simulink model "NL_Simulation"  (R2018b)
settings: Solver=VariableStepAuto  StartTime=0.0  StopTime=12.4  FixedStep=0.01
model workspace: external: MAT-File /home/abhineet/Research/Nonlinear_Model/Simulation_6dof/NL_Sim/setup_NL.mat (data not in the file)
values from neighbouring files (symbols this model uses):
  StateVals = SetInitial(Vinf,AeroType)    [setup_NL.m]
undefined symbols (not defined in the file or in its folder): AC, Mass
libraries: Tools_6dofSimulation x24, aerolibasang x3, dspmathops x3, shared6dofsys x2, shared6dof x2, aerolibatmos2 x1, sharedtransform x1, sharedutil x1
(part 1 of 2)
settings Model: SimulationMode=rapid-accelerator  Creator=abhineet  LastModifiedBy=abhineet
settings DataIOCC: ExternalInput=untitled.getElement('Throttle'),[]  InitialState=getstatestruct(Op_Pur)  SaveOutput=off  SignalLogging=off  DSMLogging=off  SaveTime=off
settings DebuggingCC: ReadBeforeWriteMsg=DisableAll  WriteAfterWriteMsg=DisableAll  WriteAfterReadMsg=DisableAll  MultiTaskDSMMsg=none  SignalLabelMismatchMsg=warning  LibraryContextMissingDiagnostic=none  StrictBusMsg=ErrorOnBusTreatedAsVector  NonBusSignalsTreatedAsBus=warning
settings ModelReferenceCC: UpdateModelReferenceTargets=IfOutOfDate
settings SFSimCC: SFSimEcho=off  SimUseLocalCustomCode=off
settings RTWCC: RTWUseLocalCustomCode=off

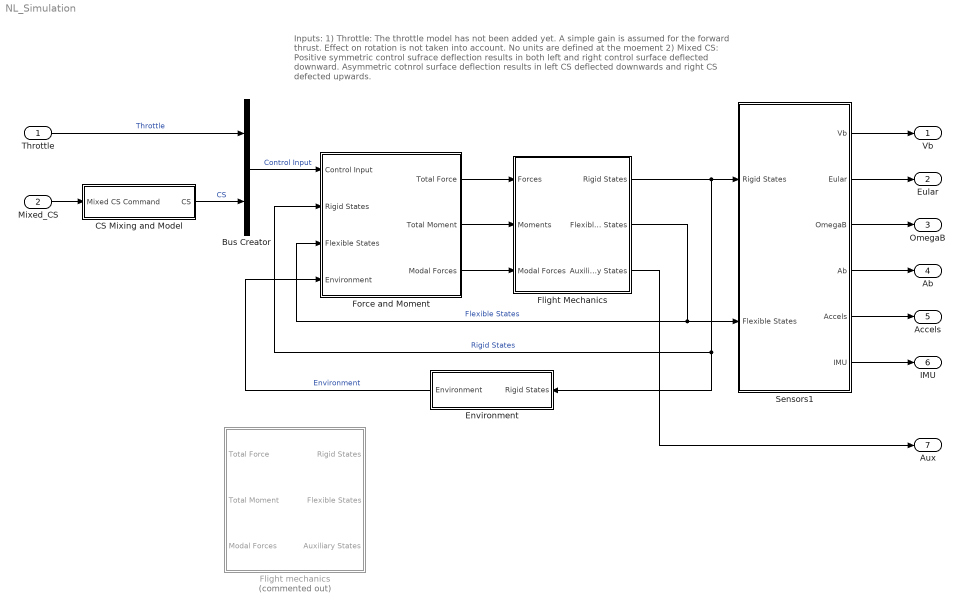
== system NL_Simulation ==
  note: Inputs:
      | 1) Throttle: The throttle model has not been added yet. A simple gain is assumed for the forward thrust.
      | 	Effect on rotation is not taken into account. No units are defined at the moement
      | 2) Mixed CS: Positive symmetric control sufrace deflection results in both left and right control surface
      | 	deflected downward. Asymmetric cotnrol surface deflection results in left CS deflected downwards
      | 	and right CS defected upwards.
  Throttle : Inport
  Mixed_CS : Inport  Port=2
  Bus Creator : BusCreator  Inputs=2
  CS Mixing and Model : Subsystem
  Environment : Subsystem
  Flight Mechanics : Subsystem  mask{units=Metric (MKS), xme_0=StateVals.Xe, Vm_0=StateVals.Vb, eul_0=StateVals.Eular, pm_0=StateVals.AngRates, mass_0=AC.MassProp.mass, inertia=AC.MassProp.inertia, xme_statename='', Vm_statename='', eul_statename='', pm_statename=''}
      mask prompts: xme_0 "Initial position in inertial axes [Xe,Ye,Ze]:"; Vm_0 "Initial velocity in body axes [U,v,w]:"; eul_0 "Initial Euler orientation [roll, pitch, yaw]:"; pm_0 "Initial body rotation rates [p,q,r]:"; mass_0 "Mass:"; xme_statename "Position: e.g., {'Xe', 'Ye', 'Ze'}"; Vm_statename "Velocity: e.g., {'U', 'v', 'w'}"; eul_statename "Euler roration angles: e.g., {'phi', 'theta', 'psi'}"; pm_statename "Body roration rates: e.g., {'p', 'q', 'r'}"
      mask TypeOptions units: Metric (MKS)
      mask DialogControl Container3 Prompt: State Names
  Flight mechanics : Subsystem  Commented=on
  "Force and Moment " : Subsystem
  Sensors1 : Subsystem
  Vb : Outport
  Eular : Outport  Port=2
  OmegaB : Outport  Port=3
  Ab : Outport  Port=4
  Accels : Outport  Port=5
  IMU : Outport  Port=6
  Aux : Outport  Port=7
  wires:
  "Force and Moment "/1(Total Force) -> Flight Mechanics/1(Forces)
  "Force and Moment "/2(Total Moment) -> Flight Mechanics/2(Moments)
  Bus Creator/1 -> "Force and Moment "/1(Control Input)  "Control Input"
  Flight Mechanics/1(Rigid States) -> Sensors1/1(Rigid States), "Force and Moment "/2(Rigid States), Environment/1(Rigid States)  "Rigid States"
  "Force and Moment "/3(Modal Forces) -> Flight Mechanics/3(Modal Forces)
  Flight Mechanics/2(Flexible States) -> Sensors1/2(Flexible States), "Force and Moment "/3(Flexible States)  "Flexible States"
  Environment/1(Environment) -> "Force and Moment "/4(Environment)  "Environment"
  CS Mixing and Model/1(CS) -> Bus Creator/2  "CS"
  Throttle/1 -> Bus Creator/1  "Throttle"
  Sensors1/3(OmegaB) -> OmegaB/1
  Sensors1/2(Eular) -> Eular/1
  Sensors1/4(Ab) -> Ab/1
  Sensors1/1(Vb) -> Vb/1
  Flight Mechanics/3(Auxiliary States) -> Aux/1
  Sensors1/6(IMU) -> IMU/1
  Sensors1/5(Accels) -> Accels/1
  Mixed_CS/1 -> CS Mixing and Model/1(Mixed CS Command)

== system NL_Simulation/CS Mixing and Model ==
  Mixed CS Command : Inport
  CS Mixing : Subsystem
  CS Model : Subsystem
  CS Model_old : Subsystem  Commented=on
  CS : Outport
  wires:
  CS Mixing/1(CS Command) -> CS Model/1(CS Command)
  CS Model/1(CS) -> CS/1
  Mixed CS Command/1 -> CS Mixing/1(Mixed CS Command)

== system NL_Simulation/Environment ==
  Rigid States : Inport
  Bus Creator : BusCreator  Inputs=1
  Bus Selector : BusSelector  OutputSignals=Xe
  COESA Atmosphere Model : aerolibatmos2/COESA Atmosphere Model  units=Metric (MKS)  spec=1976 COESA-extended U.S. Standard Atmosphere  model=Profile  profile_var=High temperature  profile_percent=1%  profile_alt=5 km (16404 ft)  envelope_var=High temperature  envelope_percent=1%  action=Warning
  Demux : Demux  Outputs=3
  Gain : Gain  Gain=-1
  Terminator{,1..4} (5 alike) : Terminator
  Environment : Outport
  wires:
  Rigid States/1 -> Bus Selector/1
  COESA Atmosphere Model/1 -> Terminator2/1
  COESA Atmosphere Model/2 -> Terminator1/1
  COESA Atmosphere Model/3 -> Terminator/1
  COESA Atmosphere Model/4 -> Bus Creator/1  "Rho"
  Bus Creator/1 -> Environment/1  "Environment"
  Bus Selector/1 -> Demux/1  "<Xe>"
  Demux/2 -> Terminator3/1
  Demux/1 -> Terminator4/1
  Demux/3 -> Gain/1  "Ze"
  Gain/1 -> COESA Atmosphere Model/1

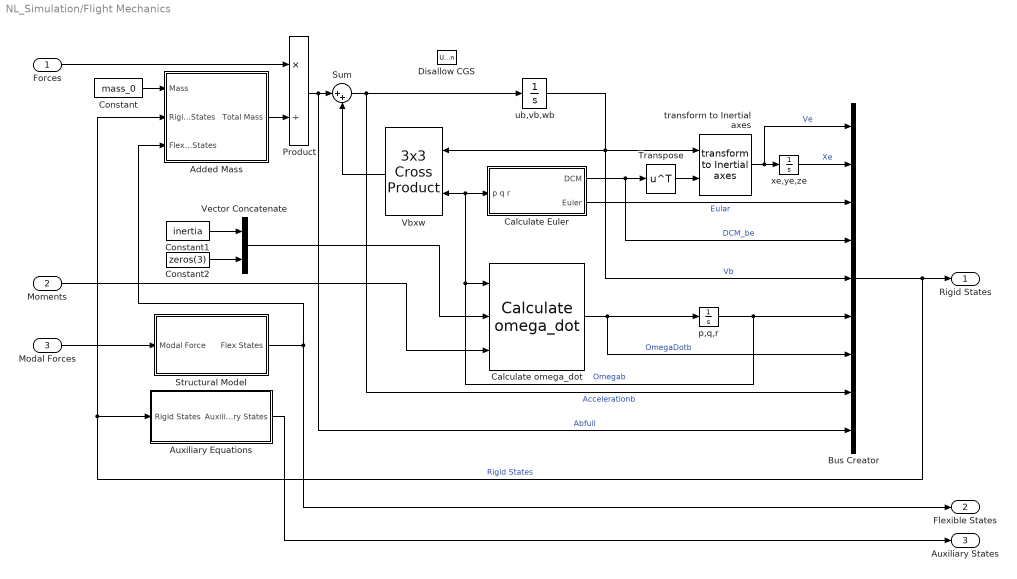
== system NL_Simulation/Flight Mechanics ==
  Forces : Inport  Unit=N  PortDimensions=3
  Moments : Inport  Port=2  Unit=N*m  PortDimensions=3
  Modal Forces : Inport  Port=3  Unit=N*m
  Added Mass : Subsystem
  "Auxiliary Equations " : Subsystem
  Bus Creator : BusCreator  Inputs=9
  Calculate Euler : Subsystem
  Calculate omega_dot : shared6dofsys/Calculate omega_dot  aMode=aMode
      settings: SourceProductName=Aerospace Blockset  SourceProductBaseCode=AE
  Constant : Constant  Value=mass_0  OutDataTypeStr=Inherit: Inherit via back propagation
  Constant1 : Constant  Value=inertia  OutDataTypeStr=Inherit: Inherit via back propagation
  Constant2 : Constant  Value=zeros(3)
  Disallow CGS : UnitConfiguration  UnitSystemsStr=English,SI,SI (extended)  AllowAllUnitSystems=off
  Product : Product  Inputs=*/  SaturateOnIntegerOverflow=on  OutDataTypeStr=Inherit: Same as first input
  Structural Model : Subsystem
  Sum : Sum  Inputs=|++  SaturateOnIntegerOverflow=on
  Transpose : Math  Operator=transpose  SaturateOnIntegerOverflow=on
  Vbxw : sharedutil/3x3 Cross Product  aMode=aMode
      settings: SourceProductBaseCode=AE
  Vector Concatenate : Concatenate  Mode=Multidimensional array
  "p,q,r " : Integrator  InitialCondition=pm_0  ContinuousStateAttributes=pm_statename
  "transform to Inertial axes " : shared6dof/6DOF (Euler Angles)/transform to Inertial axes   SystemSampleTime=-1
      settings: SourceProductName=Aerospace Blockset  SourceProductBaseCode=AE
  ub,vb,wb : Integrator  InitialCondition=Vm_0  ContinuousStateAttributes=Vm_statename
  xe,ye,ze : Integrator  InitialCondition=xme_0  ContinuousStateAttributes=xme_statename
  Rigid States : Outport
  Flexible States : Outport  Port=2
  Auxiliary States : Outport  Port=3
  wires:
  Constant/1 -> Added Mass/1(Mass)
  Vbxw/1 -> Sum/2
  Vector Concatenate/1 -> Calculate omega_dot/2
  Forces/1 -> Product/1
  Product/1 -> Bus Creator/9, Sum/1  "Abfull"
  Transpose/1 -> "transform to Inertial axes "/2
  Moments/1 -> Calculate omega_dot/3
  Added Mass/1(Total Mass) -> Product/2
  "transform to Inertial axes "/1 -> Bus Creator/1, xe,ye,ze/1  "Ve"
  xe,ye,ze/1 -> Bus Creator/2  "Xe"
  "p,q,r "/1 -> Calculate Euler/1("p q r "), Vbxw/2, Calculate omega_dot/1, Bus Creator/6  "Omegab"
  Calculate Euler/2(Euler) -> Bus Creator/3  "Eular"
  ub,vb,wb/1 -> Bus Creator/5, Vbxw/1, "transform to Inertial axes "/1  "Vb"
  Calculate Euler/1(DCM) -> Bus Creator/4, Transpose/1  "DCM_be"
  Calculate omega_dot/1 -> "p,q,r "/1, Bus Creator/7  "OmegaDotb"
  Sum/1 -> ub,vb,wb/1, Bus Creator/8  "Accelerationb"
  Bus Creator/1 -> Rigid States/1, "Auxiliary Equations "/1(Rigid States), Added Mass/2(Rigid States)  "Rigid States"
  Modal Forces/1 -> Structural Model/1(Modal Force)
  Structural Model/1(Flex States) -> Flexible States/1, Added Mass/3(Flexible States)
  Constant2/1 -> Vector Concatenate/2
  Constant1/1 -> Vector Concatenate/1
  "Auxiliary Equations "/1(Auxiliary States) -> Auxiliary States/1

== system NL_Simulation/Flight mechanics ==
  Total Force : Inport
  Total Moment : Inport  Port=2
  Modal Forces : Inport  Port=3
  "Auxiliary Equations " : Subsystem
  Subsystem1 : Subsystem  Commented=on
  Subsystem2 : Subsystem  Commented=on
  Rigid States : Outport
  Flexible States : Outport  Port=2
  Auxiliary States : Outport  Port=3
  wires:
  Total Moment/1 -> ?
  Total Force/1 -> ?
  ? -> "Auxiliary Equations "/1(Rigid States), Rigid States/1
  "Auxiliary Equations "/1(Auxiliary States) -> Auxiliary States/1
  Modal Forces/1 -> ?
  ? -> Flexible States/1

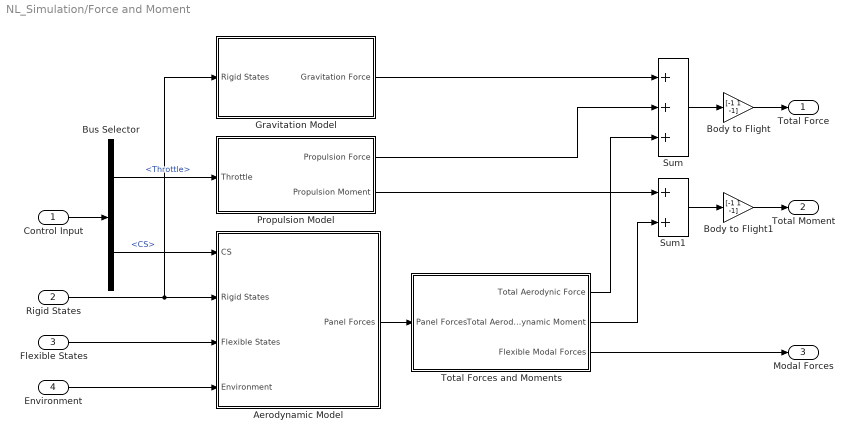
== system NL_Simulation/Force and Moment  ==
  Control Input : Inport
  Rigid States : Inport  Port=2
  Flexible States : Inport  Port=3
  Environment : Inport  Port=4
  Aerodynamic Model : Subsystem
  Body to Flight : Gain  Gain=[-1 1 -1]
  Body to Flight1 : Gain  Gain=[-1 1 -1]
  Bus Selector : BusSelector  OutputSignals=Throttle,CS
  Gravitation Model : Subsystem
  Propulsion Model : Subsystem
  Sum : Sum  Inputs=+++
  Sum1 : Sum
  Total Forces and Moments : Subsystem
  Total Force : Outport
  Total Moment : Outport  Port=2
  Modal Forces : Outport  Port=3
  wires:
  Control Input/1 -> Bus Selector/1
  Bus Selector/1 -> Propulsion Model/1(Throttle)  "<Throttle>"
  Bus Selector/2 -> Aerodynamic Model/1(CS)  "<CS>"
  Rigid States/1 -> Aerodynamic Model/2(Rigid States), Gravitation Model/1(Rigid States)
  Flexible States/1 -> Aerodynamic Model/3(" Flexible States")
  Sum/1 -> Body to Flight/1
  Environment/1 -> Aerodynamic Model/4(Environment)
  Total Forces and Moments/1(Total Aerodynic Force) -> Sum/3
  Total Forces and Moments/2(Total Aerodynamic Moment) -> Sum1/2
  Aerodynamic Model/1(Panel Forces) -> Total Forces and Moments/1(Panel Forces)
  Propulsion Model/1(Propulsion Force) -> Sum/2
  Gravitation Model/1(Gravitation Force) -> Sum/1
  Propulsion Model/2(Propulsion Moment) -> Sum1/1
  Sum1/1 -> Body to Flight1/1
  Body to Flight/1 -> Total Force/1
  Body to Flight1/1 -> Total Moment/1
  Total Forces and Moments/3(Flexible Modal Forces) -> Modal Forces/1

== system NL_Simulation/Sensors1 ==
  Rigid States : Inport
  Flexible States : Inport  Port=2
  Accelerometer Rigid : Subsystem  Commented=on
  Accelerometers : Subsystem
  Bus Selector : BusSelector  OutputSignals=Vb,Eular,Omegab,Accelerationb
  IMUs : Subsystem
  Sensors : Subsystem  Commented=on
  Vb : Outport
  Eular : Outport  Port=2
  OmegaB : Outport  Port=3
  Ab : Outport  Port=4
  Accels : Outport  Port=5
  IMU : Outport  Port=6
  wires:
  Rigid States/1 -> IMUs/1(Rigid States), Accelerometers/1(Rigid States), Bus Selector/1
  Flexible States/1 -> IMUs/2(Flexible States), Accelerometers/2(Flexible States)
  Bus Selector/3 -> OmegaB/1  "<Omegab>"
  Bus Selector/2 -> Eular/1  "<Eular>"
  Bus Selector/4 -> Ab/1  "<Accelerationb>"
  Bus Selector/1 -> Vb/1  "<Vb>"
  Accelerometers/1(Accels) -> Accels/1
  IMUs/1(IMU) -> IMU/1

== system NL_Simulation/CS Mixing and Model/CS Mixing ==
  Mixed CS Command : Inport
  Demux : Demux  Outputs=8
  Mux : Mux  Inputs=8
  Sum{,1..3} (4 alike) : Sum  Inputs=|++
  Sum{4..7} (4 alike) : Sum  Inputs=+-|
  CS Command : Outport
  wires:
  Demux/7 -> Sum6/2, Sum2/2  "Asym 3"
  Sum/1 -> Mux/1  "L1"
  Sum4/1 -> Mux/5  "R1"
  Sum7/1 -> Mux/8  "R4"
  Demux/8 -> Sum7/2, Sum3/2  "Asym 4"
  Demux/2 -> Sum5/1, Sum1/1  "Sym 2"
  Demux/1 -> Sum4/1, Sum/1  "Sym 1"
  Demux/4 -> Sum7/1, Sum3/1  "Sym 4"
  Sum1/1 -> Mux/2  "L2"
  Demux/5 -> Sum4/2, Sum/2  "Asym 1"
  Sum2/1 -> Mux/3  "L3"
  Demux/3 -> Sum6/1, Sum2/1  "Sym 3"
  Sum5/1 -> Mux/6  "R2"
  Sum6/1 -> Mux/7  "R3"
  Demux/6 -> Sum5/2, Sum1/2  "Asym 2"
  Mixed CS Command/1 -> Demux/1
  Sum3/1 -> Mux/4  "L4"
  Mux/1 -> CS Command/1

== system NL_Simulation/CS Mixing and Model/CS Model ==
  note: A second order actuator model is used: b/(s^2 + as + b)
  CS Command : Inport
  Actuator_a : Gain  Gain=AC.Actuator.a
  Actuator_b : Gain  Gain=AC.Actuator.b
  Bus Creator : BusCreator  Inputs=2
  CS Pos : Integrator  InitialCondition=StateVals.CSPos
  CS Vel : Integrator  InitialCondition=StateVals.CSVel
  Scope : Scope
  Sum : Sum  Inputs=|+-
  Sum1 : Sum  Inputs=|+-
  CS : Outport
  wires:
  CS Pos/1 -> Sum/2, Bus Creator/1  "CS Pos"
  CS Vel/1 -> Scope/1, CS Pos/1, Actuator_a/1, Bus Creator/2  "CS Vel"
  Actuator_b/1 -> Sum1/1
  CS Command/1 -> Sum/1
  Sum/1 -> Actuator_b/1
  Actuator_a/1 -> Sum1/2
  Sum1/1 -> CS Vel/1
  Bus Creator/1 -> CS/1

== system NL_Simulation/CS Mixing and Model/CS Model_old ==
  CS Command : Inport
  Bus Creator : BusCreator  Inputs=2
  CS Pos : Integrator  InitialCondition=StateVals.CSPos
  Gain : Gain  Gain=AC.CS.CSTau
  Sum : Sum  Inputs=|+-
  CS : Outport
  wires:
  CS Command/1 -> Sum/1
  Sum/1 -> Gain/1
  Gain/1 -> Bus Creator/2, CS Pos/1  "CS Vel"
  CS Pos/1 -> Bus Creator/1, Sum/2  "CS Pos"
  Bus Creator/1 -> CS/1  "CS"

== system NL_Simulation/Flight Mechanics/Added Mass ==
  Mass : Inport
  Rigid States : Inport  Port=2
  Flexible States : Inport  Port=3
  Mux : Mux  Inputs=3
  Subsystem3 : Subsystem  Commented=on
  Sum1 : Sum
  Sum2 : Sum
  Sum3 : Sum
  Total Mass : Outport
  wires:
  Mass/1 -> Sum3/1, Sum2/1, Sum1/1
  Subsystem3/1(Mx) -> Sum1/2
  Subsystem3/2(My) -> Sum2/2
  Subsystem3/3(Mz) -> Sum3/2
  Sum1/1 -> Mux/1
  Sum2/1 -> Mux/2
  Sum3/1 -> Mux/3
  Mux/1 -> Total Mass/1
  Rigid States/1 -> Subsystem3/1(Rigid States)
  Flexible States/1 -> Subsystem3/2(Flexible States)

== system NL_Simulation/Flight Mechanics/Auxiliary Equations  ==
  Rigid States : Inport
  Bus Creator1 : BusCreator  Inputs=3
  Bus Selector : BusSelector  OutputSignals=Vb
  "Incidence, Sideslip, & Airspeed" : aerolibasang/Incidence, Sideslip, & Airspeed
      settings: SourceProductName=Aerospace Blockset
  Auxiliary States : Outport
  wires:
  Bus Creator1/1 -> Auxiliary States/1  "Wind Parameters"
  "Incidence, Sideslip, & Airspeed"/3 -> Bus Creator1/3  "vinf"
  "Incidence, Sideslip, & Airspeed"/2 -> Bus Creator1/2  "beta"
  "Incidence, Sideslip, & Airspeed"/1 -> Bus Creator1/1  "alpha"
  Rigid States/1 -> Bus Selector/1  "Rigid States"
  Bus Selector/1 -> "Incidence, Sideslip, & Airspeed"/1  "<Vb>"

== system NL_Simulation/Flight Mechanics/Calculate Euler ==
  "p q r " : Inport
  Rotation Angles to Direction Cosine Matrix : sharedtransform/Rotation Angles to Direction Cosine Matrix  rotationOrder=ZYX  aMode=aMode
      settings: SourceProductBaseCode=AE
  Selector : Selector  InputPortWidth=3  IndexOptions=Index vector (dialog)  Indices=[3 2 1]  OutputSizes=1
  phi theta psi : Integrator  InitialCondition=eul_0  WrapState=on  ContinuousStateAttributes=eul_statename
  phidot thetadot psidot : shared6dofsys/DCM & Euler Angles (Euler)/phidot thetadot psidot  SystemSampleTime=-1
      settings: SourceProductName=Aerospace Blockset  SourceProductBaseCode=AE
  DCM : Outport
  Euler : Outport  Port=2
  wires:
  phidot thetadot psidot/1 -> phi theta psi/1
  "p q r "/1 -> phidot thetadot psidot/1
  phi theta psi/1 -> Selector/1, phidot thetadot psidot/2, Euler/1
  Rotation Angles to Direction Cosine Matrix/1 -> DCM/1
  Selector/1 -> Rotation Angles to Direction Cosine Matrix/1

== system NL_Simulation/Flight Mechanics/Structural Model ==
  Modal Force : Inport
  Bus Creator : BusCreator  Inputs=3
  Damping : Gain  Gain=AC.ModalStruc.Damping
  Eta : Integrator  InitialCondition=StateVals.Eta
  Etadot : Integrator  InitialCondition=StateVals.EtaDot
  InverseMass : Gain  Gain=AC.ModalStruc.InvMass
  Stiffness : Gain  Gain=AC.ModalStruc.Stiffness
  Sum : Sum  Inputs=|+-
  Sum1 : Sum  Inputs=|+-
  Flex States : Outport
  wires:
  InverseMass/1 -> Bus Creator/3, Etadot/1  "EtaFlexdotdot"
  Etadot/1 -> Damping/1, Bus Creator/2, Eta/1  "EtaFlexdot"
  Damping/1 -> Sum/2
  Eta/1 -> Bus Creator/1, Stiffness/1  "EtaFlex"
  Sum/1 -> InverseMass/1
  Sum1/1 -> Sum/1
  Modal Force/1 -> Sum1/1
  Bus Creator/1 -> Flex States/1  "Flex States"
  Stiffness/1 -> Sum1/2

== system NL_Simulation/Flight mechanics/Auxiliary Equations  ==
  Rigid States : Inport
  Bus Creator1 : BusCreator  Inputs=3
  Bus Selector : BusSelector  OutputSignals=Vb
  "Incidence, Sideslip, & Airspeed" : aerolibasang/Incidence, Sideslip, & Airspeed
      settings: SourceProductName=Aerospace Blockset
  Auxiliary States : Outport
  wires:
  Bus Creator1/1 -> Auxiliary States/1  "Wind Parameters"
  "Incidence, Sideslip, & Airspeed"/3 -> Bus Creator1/3  "vinf"
  "Incidence, Sideslip, & Airspeed"/2 -> Bus Creator1/2  "beta"
  "Incidence, Sideslip, & Airspeed"/1 -> Bus Creator1/1  "alpha"
  Rigid States/1 -> Bus Selector/1  "Rigid States"
  Bus Selector/1 -> "Incidence, Sideslip, & Airspeed"/1  "<Vb>"

== system NL_Simulation/Flight mechanics/Subsystem1 ==
  In1 : Inport
  In2 : Inport  Port=2
  In3 : Inport  Port=3
  6DOF : shared6dof/6DOF (Euler Angles)  units=Metric (MKS)  mtype=Fixed  rep=Euler Angles  xme_0=StateVals.Xe  Vm_0=StateVals.Vb  eul_0=StateVals.Eular  pm_0=StateVals.AngRates  mass_0=AC.MassProp.mass  mass_e=0.5  mass_f=2.0  inertia=AC.MassProp.inertia  inertia_e=eye(3)  inertia_f=2*eye(3)  k_quat=1.0  vre_flag=on  abi_flag=off  aMode=0  xme_statename=''  Vm_statename=''  eul_statename=''  quat_statename=''  pm_statename=''  mass_statename=''
      settings: SourceProductBaseCode=AE
  "Auxiliary Equations " : Subsystem
  Bus Creator : BusCreator  Inputs=8
  Structural Model : Subsystem
  Rigid States : Outport
  Flexible States : Outport  Port=2
  Auxiliary States : Outport  Port=3
  wires:
  6DOF/3 -> Bus Creator/3  "Eular"
  "Auxiliary Equations "/1(Auxiliary States) -> Auxiliary States/1
  6DOF/4 -> Bus Creator/4  "DCM_be"
  6DOF/5 -> Bus Creator/5  "Vb"
  6DOF/6 -> Bus Creator/6  "Omegab"
  In1/1 -> 6DOF/1
  In2/1 -> 6DOF/2
  In3/1 -> Structural Model/1(Modal Force)
  Bus Creator/1 -> Rigid States/1, "Auxiliary Equations "/1(Rigid States)  "Rigid States"
  Structural Model/1(Flex States) -> Flexible States/1
  6DOF/2 -> Bus Creator/2  "Xe"
  6DOF/1 -> Bus Creator/1  "Ve"
  6DOF/7 -> Bus Creator/7  "OmegaDotb"
  6DOF/8 -> Bus Creator/8  "Accelerationb"

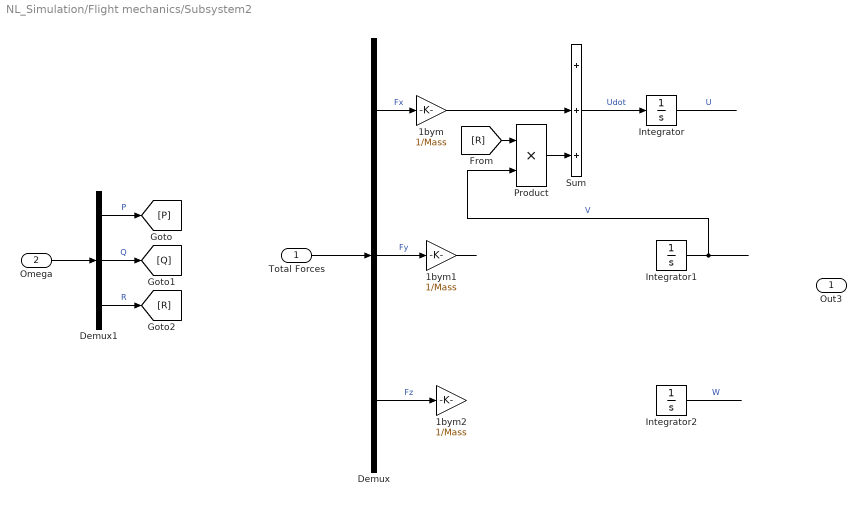
== system NL_Simulation/Flight mechanics/Subsystem2 ==
  Total Forces : Inport
  Omega : Inport  Port=2
  1bym : Gain  Gain=1/Mass
  1bym1 : Gain  Gain=1/Mass
  1bym2 : Gain  Gain=1/Mass
  Demux : Demux  Outputs=3
  Demux1 : Demux  Outputs=3
  Integrator : Integrator
  Integrator1 : Integrator
  Integrator2 : Integrator
  Product : Product
  Sum : Sum  Inputs=+++
  Out3 : Outport
  wires:
  Product/1 -> Sum/3
  1bym1/1 -> ?
  Demux/1 -> 1bym/1  "Fx"
  Demux1/3 -> [R]  "R"
  Omega/1 -> Demux1/1
  Demux/2 -> 1bym1/1  "Fy"
  Integrator/1 -> ?  "U"
  Demux1/2 -> [Q]  "Q"
  Total Forces/1 -> Demux/1
  1bym/1 -> Sum/2
  Demux1/1 -> [P]  "P"
  Sum/1 -> Integrator/1  "Udot"
  Demux/3 -> 1bym2/1  "Fz"
  Integrator1/1 -> Product/2  "V"
  ? -> Integrator1/1  "Vdot"
  ? -> Integrator2/1  "Wdot"
  Integrator2/1 -> ?  "W"
  [R] -> Product/1

== system NL_Simulation/Force and Moment /Aerodynamic Model ==
  CS : Inport
  Rigid States : Inport  Port=2
  " Flexible States" : Inport  Port=3
  Environment : Inport  Port=4
  Steady Aerodynamics : Subsystem
  Sum : Sum
  Unsteady Aerodynamics : Subsystem  Commented=on
  Panel Forces : Outport
  wires:
  CS/1 -> Steady Aerodynamics/1(CS)
  Rigid States/1 -> Unsteady Aerodynamics/1(Rigid States), Steady Aerodynamics/2(Rigid States)
  " Flexible States"/1 -> Unsteady Aerodynamics/2(Flexible States), Steady Aerodynamics/3(Flexible States)
  Environment/1 -> Steady Aerodynamics/4(Environment)
  Steady Aerodynamics/1(Total Steady Forces) -> Sum/1
  Sum/1 -> Panel Forces/1
  Unsteady Aerodynamics/1(Total Unsteady Forces) -> Sum/2

== system NL_Simulation/Force and Moment /Gravitation Model ==
  note: Gravitational force is first calculated in body fixed, flight dynamics axes and then converted to Aerodynamic Axes
  Rigid States : Inport
  Bus Selector : BusSelector  OutputSignals=DCM_be
  Constant : Constant  Value=0
  Flight Dynamics to Aero Axes : Gain  Gain=[-1 1 -1]
  Mass : Constant  Value=AC.MassProp.mass
  Mux : Mux  Inputs=3
  Product1 : Product
  Product2 : Product  Multiplication=Matrix(*)
  Reshape : Reshape  OutputDimensionality=Column vector (2-D)
  Reshape1 : Reshape
  g : Constant  Value=9.81
  Gravitation Force : Outport
  wires:
  Rigid States/1 -> Bus Selector/1
  Bus Selector/1 -> Product2/1  "<DCM_be>"
  Mass/1 -> Product1/2
  g/1 -> Product1/1
  Flight Dynamics to Aero Axes/1 -> Gravitation Force/1
  Product2/1 -> Reshape1/1
  Constant/1 -> Mux/2, Mux/1
  Product1/1 -> Mux/3  "mg"
  Mux/1 -> Reshape/1
  Reshape/1 -> Product2/2
  Reshape1/1 -> Flight Dynamics to Aero Axes/1

== system NL_Simulation/Force and Moment /Propulsion Model ==
  note: Propulsion forces and moments are calculated in Aerodynamic Axes directly
  Throttle : Inport
  Gain : Gain  Gain=[-100 0 0]
  Gain1 : Gain  Gain=[0 0 0]
  Propulsion Force : Outport
  Propulsion Moment : Outport  Port=2
  wires:
  Gain/1 -> Propulsion Force/1
  Throttle/1 -> Gain1/1, Gain/1
  Gain1/1 -> Propulsion Moment/1

== system NL_Simulation/Force and Moment /Total Forces and Moments ==
  Panel Forces : Inport
  Constant1 : Constant  Value=AC.Aero.VLMData.grid.r_cgvortex
  MATLAB Function : MATLAB Function  TreatAsAtomicUnit=on
  RB Mode Tranlation : Gain  Gain=AC.ModalStruc.Phif_aero_trans'  Multiplication=Matrix(K*u)
  Reshape : Reshape
  Reshape1 : Reshape
  Sum : Sum  Inputs=+  CollapseMode=Specified dimension  CollapseDim=2
  Total Aerodynic Force : Outport
  Total Aerodynamic Moment : Outport  Port=2
  Flexible Modal Forces : Outport  Port=3
  wires:
  MATLAB Function/1(SumRcrossF) -> Total Aerodynamic Moment/1
  RB Mode Tranlation/1 -> Flexible Modal Forces/1
  Reshape/1 -> RB Mode Tranlation/1
  Panel Forces/1 -> Reshape/1, MATLAB Function/2(F), Sum/1
  Constant1/1 -> MATLAB Function/1(R)
  Sum/1 -> Reshape1/1
  Reshape1/1 -> Total Aerodynic Force/1

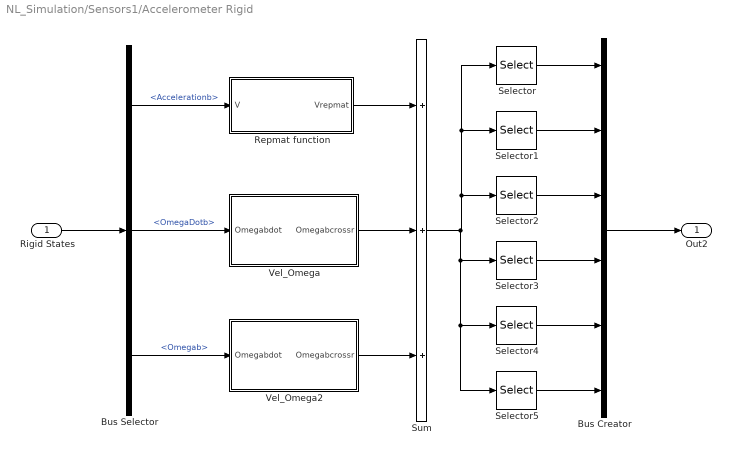
== system NL_Simulation/Sensors1/Accelerometer Rigid ==
  Rigid States : Inport
  Bus Creator : BusCreator  Inputs=6
  Bus Selector : BusSelector  OutputSignals=Accelerationb,OmegaDotb,Omegab
  Repmat function : MATLAB Function  TreatAsAtomicUnit=on  mask{NumSensors=AC.SensorData.NumSensors}
      mask prompts: NumSensors "Number of Sensors"
      mask init:
      | % NumPanels = 888;
  Selector : Selector  NumberOfDimensions=2  InputPortWidth=2  IndexOptions=Index vector (dialog),Index vector (dialog)  Indices=3,1  OutputSizes=1,1
  Selector1 : Selector  NumberOfDimensions=2  InputPortWidth=2  IndexOptions=Index vector (dialog),Index vector (dialog)  Indices=3,2  OutputSizes=1,1
  Selector2 : Selector  NumberOfDimensions=2  InputPortWidth=2  IndexOptions=Index vector (dialog),Index vector (dialog)  Indices=3,3  OutputSizes=1,1
  Selector3 : Selector  NumberOfDimensions=2  InputPortWidth=2  IndexOptions=Index vector (dialog),Index vector (dialog)  Indices=3,4  OutputSizes=1,1
  Selector4 : Selector  NumberOfDimensions=2  InputPortWidth=2  IndexOptions=Index vector (dialog),Index vector (dialog)  Indices=3,5  OutputSizes=1,1
  Selector5 : Selector  NumberOfDimensions=2  InputPortWidth=2  IndexOptions=Index vector (dialog),Index vector (dialog)  Indices=3,6  OutputSizes=1,1
  Sum : Sum  Inputs=+++
  Vel_Omega : Subsystem
  Vel_Omega2 : Subsystem
  Out2 : Outport
  wires:
  Rigid States/1 -> Bus Selector/1
  Bus Selector/1 -> Repmat function/1(V)  "<Accelerationb>"
  Bus Selector/2 -> Vel_Omega/1(Omegabdot)  "<OmegaDotb>"
  Vel_Omega/1(Omegabcrossr) -> Sum/2
  Repmat function/1(Vrepmat) -> Sum/1
  Bus Selector/3 -> Vel_Omega2/1(Omegabdot)  "<Omegab>"
  Vel_Omega2/1(Omegabcrossr) -> Sum/3
  Sum/1 -> Selector4/1, Selector5/1, Selector3/1, Selector/1, Selector1/1, Selector2/1
  Selector/1 -> Bus Creator/1
  Selector1/1 -> Bus Creator/2
  Selector2/1 -> Bus Creator/3
  Selector3/1 -> Bus Creator/4
  Selector5/1 -> Bus Creator/6
  Selector4/1 -> Bus Creator/5
  Bus Creator/1 -> Out2/1

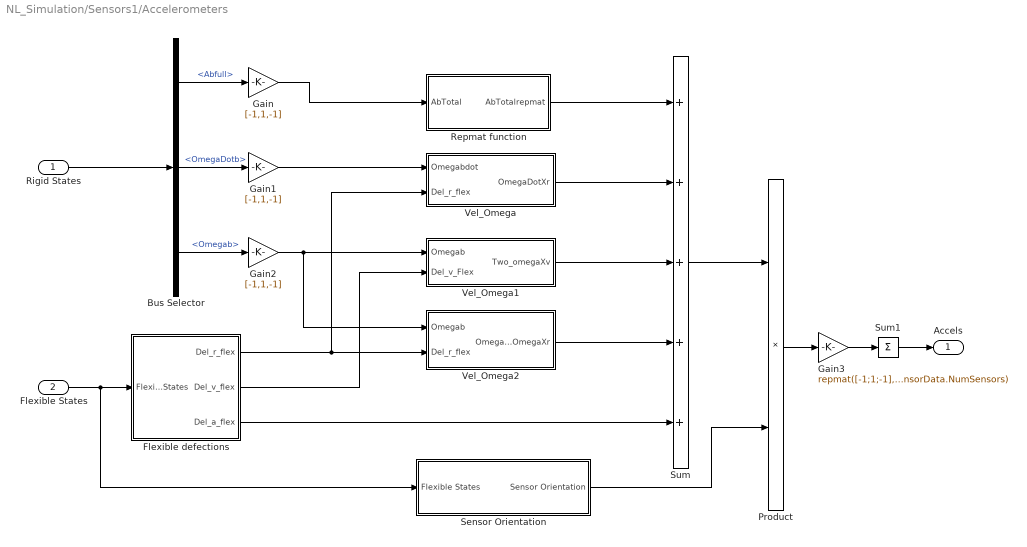
== system NL_Simulation/Sensors1/Accelerometers ==
  Rigid States : Inport
  Flexible States : Inport  Port=2
  Bus Selector : BusSelector  OutputSignals=Abfull,OmegaDotb,Omegab
  Flexible defections : Subsystem
  Gain : Gain  Gain=[-1,1,-1]
  Gain1 : Gain  Gain=[-1,1,-1]
  Gain2 : Gain  Gain=[-1,1,-1]
  Gain3 : Gain  Gain=repmat([-1;1;-1],1,AC.SensorData.NumSensors)
  Product : Product
  Repmat function : MATLAB Function  TreatAsAtomicUnit=on  mask{NumSensors=AC.SensorData.NumSensors}
      mask prompts: NumSensors "Number of Sensors"
      mask init:
      | % NumPanels = 888;
  Sensor Orientation : Subsystem
  Sum : Sum  Inputs=+++++
  Sum1 : Sum  Inputs=+  CollapseMode=Specified dimension
  Vel_Omega : Subsystem
  Vel_Omega1 : Subsystem
  Vel_Omega2 : Subsystem
  Accels : Outport
  wires:
  Rigid States/1 -> Bus Selector/1
  Bus Selector/1 -> Gain/1  "<Abfull>"
  Vel_Omega/1(OmegaDotXr) -> Sum/2
  Vel_Omega2/1(OmegaXOmegaXr) -> Sum/4
  Flexible States/1 -> Sensor Orientation/1(Flexible States), Flexible defections/1(Flexible States)
  Sensor Orientation/1(Sensor Orientation) -> Product/2
  Product/1 -> Gain3/1
  Sum/1 -> Product/1
  Sum1/1 -> Accels/1
  Bus Selector/2 -> Gain1/1  "<OmegaDotb>"
  Bus Selector/3 -> Gain2/1  "<Omegab>"
  Flexible defections/3(Del_a_flex) -> Sum/5
  Repmat function/1(AbTotalrepmat) -> Sum/1
  Flexible defections/1(Del_r_flex) -> Vel_Omega2/2(Del_r_flex), Vel_Omega/2(Del_r_flex)
  Flexible defections/2(Del_v_flex) -> Vel_Omega1/2(Del_v_Flex)
  Vel_Omega1/1(Two_omegaXv) -> Sum/3
  Gain/1 -> Repmat function/1(AbTotal)
  Gain1/1 -> Vel_Omega/1(Omegabdot)
  Gain2/1 -> Vel_Omega2/1(Omegab), Vel_Omega1/1(Omegab)
  Gain3/1 -> Sum1/1

== system NL_Simulation/Sensors1/IMUs ==
  Rigid States : Inport
  Flexible States : Inport  Port=2
  Bus Selector : BusSelector  OutputSignals=Omegab
  Bus Selector1 : BusSelector  OutputSignals=EtaFlexdot
  Gain : Gain  Gain=AC.ModalStruc.Phif_aero_sensor_Rot  Multiplication=Matrix(K*u)
  Gain1 : Gain  Gain=[-1,1,-1]
  Gain2 : Gain  Gain=repmat([-1;1;-1],1,AC.SensorData.NumSensors)
  Repmat function : MATLAB Function  TreatAsAtomicUnit=on  mask{NumSensors=AC.SensorData.NumSensors}
      mask prompts: NumSensors "Number of Sensors"
      mask init:
      | % NumPanels = 888;
  Reshape : Reshape  OutputDimensionality=Customize  OutputDimensions=[3,AC.SensorData.NumSensors]
  Sum : Sum
  IMU : Outport
  wires:
  Rigid States/1 -> Bus Selector/1
  Flexible States/1 -> Bus Selector1/1
  Bus Selector1/1 -> Gain/1  "<EtaFlexdot>"
  Bus Selector/1 -> Gain1/1  "<Omegab>"
  Gain/1 -> Reshape/1
  Repmat function/1(Vrepmat) -> Sum/1
  Reshape/1 -> Sum/2
  Sum/1 -> Gain2/1
  Gain1/1 -> Repmat function/1(V)
  Gain2/1 -> IMU/1

== system NL_Simulation/Sensors1/Sensors ==
  Rigid States : Inport
  Flexible States : Inport  Port=2
  Accelerometer Rigid : Subsystem  Commented=on
  Accelerometers : Subsystem
  Bus Selector : BusSelector  OutputSignals=Vb,Eular,Omegab,Accelerationb
  IMUs : Subsystem
  Vb : Outport
  Eular : Outport  Port=2
  OmegaB : Outport  Port=3
  Ab : Outport  Port=4
  Accels : Outport  Port=5
  Accels_zcomp : Outport  Port=6
  IMU : Outport  Port=7
  wires:
  Rigid States/1 -> IMUs/1(Rigid States), Accelerometers/1(Rigid States), Bus Selector/1
  Flexible States/1 -> IMUs/2(Flexible States), Accelerometers/2(Flexible States)
  Bus Selector/3 -> OmegaB/1  "<Omegab>"
  Bus Selector/2 -> Eular/1  "<Eular>"
  Accelerometers/2(Accels_ZComp) -> Accels_zcomp/1
  Bus Selector/4 -> Ab/1  "<Accelerationb>"
  Bus Selector/1 -> Vb/1  "<Vb>"
  Accelerometers/1(Accels) -> Accels/1
  IMUs/1(IMU) -> IMU/1

== system NL_Simulation/Flight Mechanics/Added Mass/Subsystem3 ==
  Rigid States : Inport
  Flexible States : Inport  Port=2
  MATLAB Function : MATLAB Function  TreatAsAtomicUnit=on
  Nhat0 : Constant  Value=AC.Aero.Nhat0
  Normal Forces : Subsystem
  Normal Wash Derivative : Subsystem
  Total Wash Derivative : Subsystem
      mask init:
      | %% All modes
      | Sys_Ab = ss(-300,1,1,0)*eye(3);
      | Sys_OmegaDotb = ss(-300,1,1,0)*eye(3);
      | Sys_FlexDotDotb = ss(-300,1,1,0)*eye(6);
  Mx : Outport
  My : Outport  Port=2
  Mz : Outport  Port=3
  wires:
  Rigid States/1 -> Normal Forces/2(Rigid States), Total Wash Derivative/1(Rigid States)
  Flexible States/1 -> Total Wash Derivative/2(Flexible States)
  Nhat0/1 -> MATLAB Function/1(nhat0)
  Normal Forces/1(Normal Forces) -> MATLAB Function/2(NormalForces)
  Normal Wash Derivative/1(Normal Wash Derivative) -> Normal Forces/1(Normal Wash Derivatives)
  Total Wash Derivative/1(Total Wash Derivatives) -> Normal Wash Derivative/1(Total Wash Derivative)

== system NL_Simulation/Flight mechanics/Subsystem1/Auxiliary Equations  ==
  Rigid States : Inport
  Bus Creator1 : BusCreator  Inputs=3
  Bus Selector : BusSelector  OutputSignals=Vb
  "Incidence, Sideslip, & Airspeed" : aerolibasang/Incidence, Sideslip, & Airspeed
      settings: SourceProductName=Aerospace Blockset
  Auxiliary States : Outport
  wires:
  Bus Creator1/1 -> Auxiliary States/1  "Wind Parameters"
  "Incidence, Sideslip, & Airspeed"/3 -> Bus Creator1/3  "vinf"
  "Incidence, Sideslip, & Airspeed"/2 -> Bus Creator1/2  "beta"
  "Incidence, Sideslip, & Airspeed"/1 -> Bus Creator1/1  "alpha"
  Rigid States/1 -> Bus Selector/1  "Rigid States"
  Bus Selector/1 -> "Incidence, Sideslip, & Airspeed"/1  "<Vb>"

== system NL_Simulation/Flight mechanics/Subsystem1/Structural Model ==
  Modal Force : Inport
  Bus Creator : BusCreator  Inputs=3
  Damping : Gain  Gain=AC.ModalStruc.Damping
  Eta : Integrator  InitialCondition=StateVals.Eta
  Etadot : Integrator  InitialCondition=StateVals.EtaDot
  InverseMass : Gain  Gain=AC.ModalStruc.InvMass
  Stiffness : Gain  Gain=AC.ModalStruc.Stiffness
  Sum : Sum  Inputs=|+-
  Sum1 : Sum  Inputs=|+-
  Flex States : Outport
  wires:
  InverseMass/1 -> Bus Creator/3, Etadot/1  "EtaFlexdotdot"
  Etadot/1 -> Damping/1, Bus Creator/2, Eta/1  "EtaFlexdot"
  Damping/1 -> Sum/2
  Eta/1 -> Bus Creator/1, Stiffness/1  "EtaFlex"
  Sum/1 -> InverseMass/1
  Sum1/1 -> Sum/1
  Modal Force/1 -> Sum1/1
  Bus Creator/1 -> Flex States/1  "Flex States"
  Stiffness/1 -> Sum1/2

== system NL_Simulation/Force and Moment /Aerodynamic Model/Steady Aerodynamics ==
  CS : Inport
  Rigid States : Inport  Port=2
  Flexible States : Inport  Port=3
  Environment : Inport  Port=4
  N_hat : Subsystem
  Normal Wash : Subsystem
  Panel Forces Calculation : Subsystem
  Total Wash : Subsystem
  Vortex Strength : Subsystem
  Total Steady Forces : Outport
  wires:
  N_hat/1(Nhat) -> Normal Wash/1(Nhat)
  Normal Wash/1(Normal Wash) -> Vortex Strength/2(Normal wash)
  Total Wash/1(Total  Wash) -> Normal Wash/2(Total Wash)
  Panel Forces Calculation/1(Panel Forces) -> Total Steady Forces/1
  Rigid States/1 -> Total Wash/1(Rigid States), Panel Forces Calculation/1(Rigid States)
  Vortex Strength/1(Gamma) -> Panel Forces Calculation/3(Gamma)
  Environment/1 -> Panel Forces Calculation/4(Environment)
  CS/1 -> N_hat/1(CS)
  Flexible States/1 -> Total Wash/2(Flexible States), Vortex Strength/1(Flexible States), Panel Forces Calculation/2(Flexible States), N_hat/2(Flexible States)

== system NL_Simulation/Force and Moment /Aerodynamic Model/Unsteady Aerodynamics ==
  Rigid States : Inport
  Flexible States : Inport  Port=2
  MATLAB Function : MATLAB Function  TreatAsAtomicUnit=on
  Nhat0 : Constant  Value=AC.Aero.Nhat0
  Normal Forces : Subsystem
  Normal Wash Derivative : Subsystem
  Total Wash Derivative : Subsystem
      mask init:
      | %% All modes
      | Sys_Ab = ss(-300,1,1,0)*eye(3);
      | Sys_OmegaDotb = ss(-300,1,1,0)*eye(3);
      | Sys_FlexDotDotb = ss(-300,1,1,0)*eye(6);
  Total Unsteady Forces : Outport
  wires:
  Rigid States/1 -> Total Wash Derivative/1(Rigid States), Normal Forces/2(Rigid States)
  Flexible States/1 -> Total Wash Derivative/2(Flexible States)
  Normal Wash Derivative/1(Normal Wash Derivative) -> Normal Forces/1(Normal Wash Derivatives)
  Nhat0/1 -> MATLAB Function/1(nhat0)
  Normal Forces/1(Normal Forces) -> MATLAB Function/2(NormalForces)
  MATLAB Function/1(TotalForces) -> Total Unsteady Forces/1
  Total Wash Derivative/1(Total Wash Derivatives) -> Normal Wash Derivative/1(Total Wash Derivative)

== system NL_Simulation/Sensors1/Accelerometer Rigid/Vel_Omega ==
  Omegabdot : Inport
  Cross Product Matrix : Tools_6dofSimulation/Cross Product Matrix  SystemSampleTime=-1
  Demux : Demux  Outputs=3
  Product : Product  Multiplication=Matrix(*)
  rcg_sensor : Constant  Value=AC.SensorData.SensorAeroGrid
  Omegabcrossr : Outport
  wires:
  Omegabdot/1 -> Demux/1
  Product/1 -> Omegabcrossr/1
  Demux/2 -> Cross Product Matrix/2  "qdot"
  Demux/3 -> Cross Product Matrix/3  "rdot"
  Cross Product Matrix/1 -> Product/1
  rcg_sensor/1 -> Product/2
  Demux/1 -> Cross Product Matrix/1  "pdot"

== system NL_Simulation/Sensors1/Accelerometer Rigid/Vel_Omega2 ==
  Omegabdot : Inport
  Cross Product Matrix : Tools_6dofSimulation/Cross Product Matrix  SystemSampleTime=-1
  Demux : Demux  Outputs=3
  Product : Product  Multiplication=Matrix(*)
  Product1 : Product  Multiplication=Matrix(*)
  rcg_sensor : Constant  Value=AC.SensorData.SensorAeroGrid
  Omegabcrossr : Outport
  wires:
  Omegabdot/1 -> Demux/1
  Demux/2 -> Cross Product Matrix/2  "qdot"
  Demux/3 -> Cross Product Matrix/3  "rdot"
  Cross Product Matrix/1 -> Product1/1, Product/1
  rcg_sensor/1 -> Product/2
  Demux/1 -> Cross Product Matrix/1  "pdot"
  Product/1 -> Product1/2
  Product1/1 -> Omegabcrossr/1

== system NL_Simulation/Sensors1/Accelerometers/Flexible defections ==
  Flexible States : Inport
  Bus Selector1 : BusSelector  OutputSignals=EtaFlex,EtaFlexdot,EtaFlexdotdot
  Gain : Gain  Commented=on  Gain=repmat([-1;1;-1],AC.SensorData.NumSensors,5)
  Phif_Translation : Constant  Value=AC.ModalStruc.Phif_aero_sensor_Trans  VectorParams1D=off
  Product1 : Product  Multiplication=Matrix(*)
  Product2 : Product  Multiplication=Matrix(*)
  Product3 : Product  Multiplication=Matrix(*)
  Reshape1 : Reshape  OutputDimensionality=Customize  OutputDimensions=[3,AC.SensorData.NumSensors]
  Reshape2 : Reshape  OutputDimensionality=Customize  OutputDimensions=[3,AC.SensorData.NumSensors]
  Reshape3 : Reshape  OutputDimensionality=Customize  OutputDimensions=[3,AC.SensorData.NumSensors]
  Del_r_flex : Outport
  Del_v_flex : Outport  Port=2
  Del_a_flex : Outport  Port=3
  wires:
  Flexible States/1 -> Bus Selector1/1
  Bus Selector1/3 -> Product3/2  "<EtaFlexdotdot>"
  Product3/1 -> Reshape3/1
  Product1/1 -> Reshape1/1
  Product2/1 -> Reshape2/1
  Bus Selector1/2 -> Product2/2  "<EtaFlexdot>"
  Bus Selector1/1 -> Product1/2  "<EtaFlex>"
  Reshape1/1 -> Del_r_flex/1
  Reshape2/1 -> Del_v_flex/1
  Reshape3/1 -> Del_a_flex/1
  Phif_Translation/1 -> Product1/1, Product2/1, Product3/1

== system NL_Simulation/Sensors1/Accelerometers/Sensor Orientation ==
  Flexible States : Inport
  Bus Selector1 : BusSelector  OutputSignals=EtaFlex
  Gain : Gain  Gain=AC.ModalStruc.Phif_aero_sensor_Rot  Multiplication=Matrix(K*u)
  Normalization : dspmathops/Normalization  NormType=2-norm  Bias=1e-10  NormOver=Each column  Dimension=1  roundingMode=Floor  overflowMode=off  accumDataTypeStr=Inherit: Same as product output  accumLastDataTypeStr=Inherit: Same as product output  outputDataTypeStr=Inherit: Same as product output  outputMin=[]  outputMax=[]  outputLastDataTypeStr=Inherit: Same as product output
      settings: SourceProductName=DSP System Toolbox
  Reshape : Reshape  OutputDimensionality=Customize  OutputDimensions=[3,AC.SensorData.NumSensors]
  SensorOrient : Constant  Value=AC.SensorData.SensorOrientation0
  Sum1 : Sum
  Sensor Orientation : Outport
  wires:
  SensorOrient/1 -> Sum1/2
  Normalization/1 -> Sensor Orientation/1
  Reshape/1 -> Sum1/1
  Flexible States/1 -> Bus Selector1/1
  Sum1/1 -> Normalization/1
  Gain/1 -> Reshape/1
  Bus Selector1/1 -> Gain/1  "<EtaFlex>"

== system NL_Simulation/Sensors1/Accelerometers/Vel_Omega ==
  Omegabdot : Inport
  Del_r_flex : Inport  Port=2
  Cross Product Matrix : Tools_6dofSimulation/Cross Product Matrix  SystemSampleTime=-1
  Demux : Demux  Outputs=3
  Product : Product  Multiplication=Matrix(*)
  Sum : Sum
  rcg_sensor : Constant  Value=AC.SensorData.SensorCG
  OmegaDotXr : Outport
  wires:
  Omegabdot/1 -> Demux/1
  Product/1 -> OmegaDotXr/1
  Demux/2 -> Cross Product Matrix/2  "qdot"
  Demux/3 -> Cross Product Matrix/3  "rdot"
  Cross Product Matrix/1 -> Product/1
  Demux/1 -> Cross Product Matrix/1  "pdot"
  rcg_sensor/1 -> Sum/1
  Del_r_flex/1 -> Sum/2
  Sum/1 -> Product/2

== system NL_Simulation/Sensors1/Accelerometers/Vel_Omega1 ==
  Omegab : Inport
  Del_v_Flex : Inport  Port=2
  Cross Product Matrix : Tools_6dofSimulation/Cross Product Matrix  SystemSampleTime=-1
  Demux : Demux  Outputs=3
  Gain : Gain  Gain=2
  Product : Product  Multiplication=Matrix(*)
  Two_omegaXv : Outport
  wires:
  Omegab/1 -> Demux/1
  Demux/2 -> Cross Product Matrix/2  "qdot"
  Demux/3 -> Cross Product Matrix/3  "rdot"
  Cross Product Matrix/1 -> Product/1
  Del_v_Flex/1 -> Product/2
  Demux/1 -> Cross Product Matrix/1  "pdot"
  Product/1 -> Gain/1
  Gain/1 -> Two_omegaXv/1

== system NL_Simulation/Sensors1/Accelerometers/Vel_Omega2 ==
  Omegab : Inport
  Del_r_flex : Inport  Port=2
  Cross Product Matrix : Tools_6dofSimulation/Cross Product Matrix  SystemSampleTime=-1
  Demux : Demux  Outputs=3
  Product : Product  Multiplication=Matrix(*)
  Product1 : Product  Multiplication=Matrix(*)
  Sum : Sum
  rcg_sensor : Constant  Value=AC.SensorData.SensorCG
  OmegaXOmegaXr : Outport
  wires:
  Omegab/1 -> Demux/1
  Demux/2 -> Cross Product Matrix/2  "qdot"
  Demux/3 -> Cross Product Matrix/3  "rdot"
  Cross Product Matrix/1 -> Product1/1, Product/1
  Demux/1 -> Cross Product Matrix/1  "pdot"
  Product/1 -> Product1/2
  Product1/1 -> OmegaXOmegaXr/1
  Sum/1 -> Product/2
  rcg_sensor/1 -> Sum/1
  Del_r_flex/1 -> Sum/2

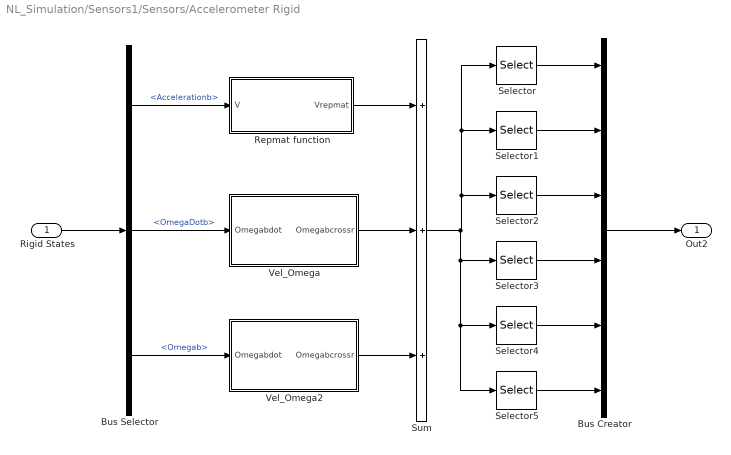
== system NL_Simulation/Sensors1/Sensors/Accelerometer Rigid ==
  Rigid States : Inport
  Bus Creator : BusCreator  Inputs=6
  Bus Selector : BusSelector  OutputSignals=Accelerationb,OmegaDotb,Omegab
  Repmat function : MATLAB Function  TreatAsAtomicUnit=on  mask{NumSensors=AC.SensorData.NumSensors}
      mask prompts: NumSensors "Number of Sensors"
      mask init:
      | % NumPanels = 888;
  Selector : Selector  NumberOfDimensions=2  InputPortWidth=2  IndexOptions=Index vector (dialog),Index vector (dialog)  Indices=3,1  OutputSizes=1,1
  Selector1 : Selector  NumberOfDimensions=2  InputPortWidth=2  IndexOptions=Index vector (dialog),Index vector (dialog)  Indices=3,2  OutputSizes=1,1
  Selector2 : Selector  NumberOfDimensions=2  InputPortWidth=2  IndexOptions=Index vector (dialog),Index vector (dialog)  Indices=3,3  OutputSizes=1,1
  Selector3 : Selector  NumberOfDimensions=2  InputPortWidth=2  IndexOptions=Index vector (dialog),Index vector (dialog)  Indices=3,4  OutputSizes=1,1
  Selector4 : Selector  NumberOfDimensions=2  InputPortWidth=2  IndexOptions=Index vector (dialog),Index vector (dialog)  Indices=3,5  OutputSizes=1,1
  Selector5 : Selector  NumberOfDimensions=2  InputPortWidth=2  IndexOptions=Index vector (dialog),Index vector (dialog)  Indices=3,6  OutputSizes=1,1
  Sum : Sum  Inputs=+++
  Vel_Omega : Subsystem
  Vel_Omega2 : Subsystem
  Out2 : Outport
  wires:
  Rigid States/1 -> Bus Selector/1
  Bus Selector/1 -> Repmat function/1(V)  "<Accelerationb>"
  Bus Selector/2 -> Vel_Omega/1(Omegabdot)  "<OmegaDotb>"
  Vel_Omega/1(Omegabcrossr) -> Sum/2
  Repmat function/1(Vrepmat) -> Sum/1
  Bus Selector/3 -> Vel_Omega2/1(Omegabdot)  "<Omegab>"
  Vel_Omega2/1(Omegabcrossr) -> Sum/3
  Sum/1 -> Selector4/1, Selector5/1, Selector3/1, Selector/1, Selector1/1, Selector2/1
  Selector/1 -> Bus Creator/1
  Selector1/1 -> Bus Creator/2
  Selector2/1 -> Bus Creator/3
  Selector3/1 -> Bus Creator/4
  Selector5/1 -> Bus Creator/6
  Selector4/1 -> Bus Creator/5
  Bus Creator/1 -> Out2/1

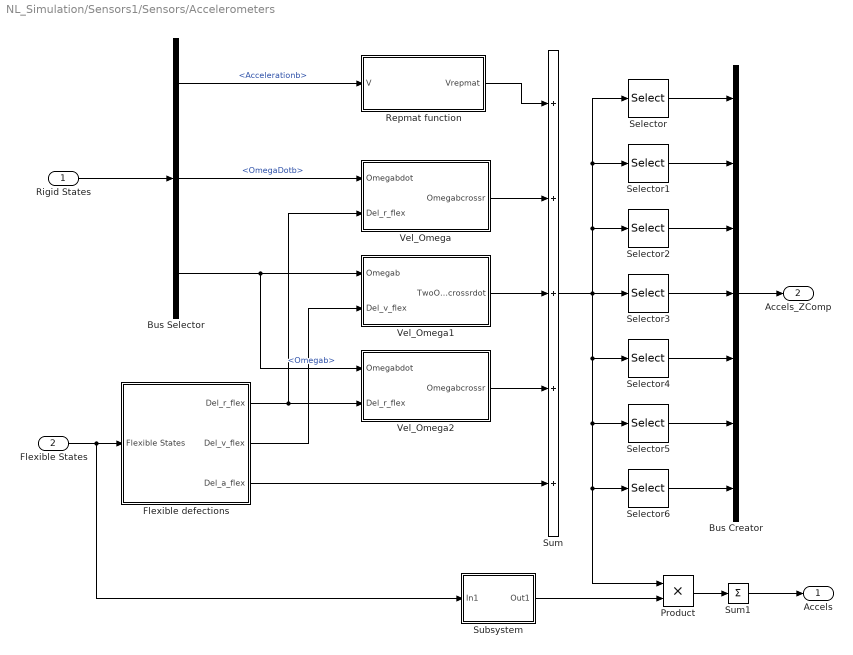
== system NL_Simulation/Sensors1/Sensors/Accelerometers ==
  Rigid States : Inport
  Flexible States : Inport  Port=2
  Bus Creator : BusCreator  Inputs=7
  Bus Selector : BusSelector  OutputSignals=Accelerationb,OmegaDotb,Omegab
  Flexible defections : Subsystem
  Product : Product
  Repmat function : MATLAB Function  TreatAsAtomicUnit=on  mask{NumSensors=AC.SensorData.NumSensors}
      mask prompts: NumSensors "Number of Sensors"
      mask init:
      | % NumPanels = 888;
  Selector : Selector  NumberOfDimensions=2  InputPortWidth=2  IndexOptions=Index vector (dialog),Index vector (dialog)  Indices=3,1  OutputSizes=1,1
  Selector1 : Selector  NumberOfDimensions=2  InputPortWidth=2  IndexOptions=Index vector (dialog),Index vector (dialog)  Indices=3,2  OutputSizes=1,1
  Selector2 : Selector  NumberOfDimensions=2  InputPortWidth=2  IndexOptions=Index vector (dialog),Index vector (dialog)  Indices=3,3  OutputSizes=1,1
  Selector3 : Selector  NumberOfDimensions=2  InputPortWidth=2  IndexOptions=Index vector (dialog),Index vector (dialog)  Indices=3,4  OutputSizes=1,1
  Selector4 : Selector  NumberOfDimensions=2  InputPortWidth=2  IndexOptions=Index vector (dialog),Index vector (dialog)  Indices=3,5  OutputSizes=1,1
  Selector5 : Selector  NumberOfDimensions=2  InputPortWidth=2  IndexOptions=Index vector (dialog),Index vector (dialog)  Indices=3,6  OutputSizes=1,1
  Selector6 : Selector  NumberOfDimensions=2  InputPortWidth=2  IndexOptions=Index vector (dialog),Index vector (dialog)  Indices=3,6  OutputSizes=1,1
  Subsystem : Subsystem
  Sum : Sum  Inputs=+++++
  Sum1 : Sum  Inputs=+  CollapseMode=Specified dimension
  Vel_Omega : Subsystem
  Vel_Omega1 : Subsystem
  Vel_Omega2 : Subsystem
  Accels : Outport
  Accels_ZComp : Outport  Port=2
  wires:
  Rigid States/1 -> Bus Selector/1
  Bus Selector/1 -> Repmat function/1(V)  "<Accelerationb>"
  Bus Selector/2 -> Vel_Omega/1(Omegabdot)  "<OmegaDotb>"
  Flexible defections/1(Del_r_flex) -> Vel_Omega2/2(Del_r_flex), Vel_Omega/2(Del_r_flex)
  Vel_Omega/1(Omegabcrossr) -> Sum/2
  Repmat function/1(Vrepmat) -> Sum/1
  Bus Selector/3 -> Vel_Omega2/1(Omegabdot), Vel_Omega1/1(Omegab)  "<Omegab>"
  Vel_Omega1/1(TwoOmegabcrossrdot) -> Sum/3
  Flexible defections/2(Del_v_flex) -> Vel_Omega1/2(Del_v_flex)
  Flexible defections/3(Del_a_flex) -> Sum/5
  Vel_Omega2/1(Omegabcrossr) -> Sum/4
  Flexible States/1 -> Subsystem/1(In1), Flexible defections/1(Flexible States)
  Subsystem/1(Out1) -> Product/2
  Product/1 -> Sum1/1
  Sum/1 -> Selector6/1, Product/1, Selector5/1, Selector4/1, Selector2/1, Selector1/1, Selector/1, Selector3/1
  Selector/1 -> Bus Creator/1
  Selector1/1 -> Bus Creator/2
  Selector2/1 -> Bus Creator/3
  Selector3/1 -> Bus Creator/4
  Selector5/1 -> Bus Creator/6
  Selector4/1 -> Bus Creator/5
  Bus Creator/1 -> Accels_ZComp/1
  Sum1/1 -> Accels/1
  Selector6/1 -> Bus Creator/7

== system NL_Simulation/Sensors1/Sensors/IMUs ==
  Rigid States : Inport
  Flexible States : Inport  Port=2
  Bus Selector : BusSelector  OutputSignals=Omegab
  Bus Selector1 : BusSelector  OutputSignals=EtaFlexdot
  Gain : Gain  Gain=AC.ModalStruc.Phif_aero_sensor_Rot  Multiplication=Matrix(K*u)
  Repmat function : MATLAB Function  TreatAsAtomicUnit=on  mask{NumSensors=AC.SensorData.NumSensors}
      mask prompts: NumSensors "Number of Sensors"
      mask init:
      | % NumPanels = 888;
  Reshape : Reshape  OutputDimensionality=Customize  OutputDimensions=[3,AC.SensorData.NumSensors]
  Sum : Sum
  IMU : Outport
  wires:
  Rigid States/1 -> Bus Selector/1
  Flexible States/1 -> Bus Selector1/1
  Bus Selector1/1 -> Gain/1  "<EtaFlexdot>"
  Bus Selector/1 -> Repmat function/1(V)  "<Omegab>"
  Gain/1 -> Reshape/1
  Repmat function/1(Vrepmat) -> Sum/1
  Reshape/1 -> Sum/2
  Sum/1 -> IMU/1

== system NL_Simulation/Flight Mechanics/Added Mass/Subsystem3/Normal Forces ==
  Normal Wash Derivatives : Inport
  Rigid States : Inport  Port=2
  Gain : Gain  Gain=AC.Aero.DLMData.A1  Multiplication=Matrix(K*u)
  Gain1 : Gain  Gain=AC.Aero.DLMData.Clag  Multiplication=Matrix(K*u)
  MACby2V : Subsystem
  Product : Product
  Subsystem1 : Subsystem
  Sum : Sum
  Normal Forces : Outport
  wires:
  Normal Wash Derivatives/1 -> Product/1
  Sum/1 -> Normal Forces/1
  Rigid States/1 -> MACby2V/1(Rigid States)
  MACby2V/1(MACby2V) -> Product/2, Subsystem1/2(b_over_V)
  Product/1 -> Subsystem1/1(Normal Wash Derivative), Gain/1
  Gain/1 -> Sum/1
  Subsystem1/1(Lag States) -> Gain1/1
  Gain1/1 -> Sum/2

== system NL_Simulation/Flight Mechanics/Added Mass/Subsystem3/Normal Wash Derivative ==
  Total Wash Derivative : Inport
  Constant : Constant  Value=AC.Aero.Nhat0
  Product : Product
  Sum : Sum  Inputs=+  CollapseMode=Specified dimension
  Transpose : Math  Operator=transpose  SaturateOnIntegerOverflow=on
  Normal Wash Derivative : Outport
  wires:
  Sum/1 -> Transpose/1
  Constant/1 -> Product/1
  Total Wash Derivative/1 -> Product/2
  Product/1 -> Sum/1
  Transpose/1 -> Normal Wash Derivative/1

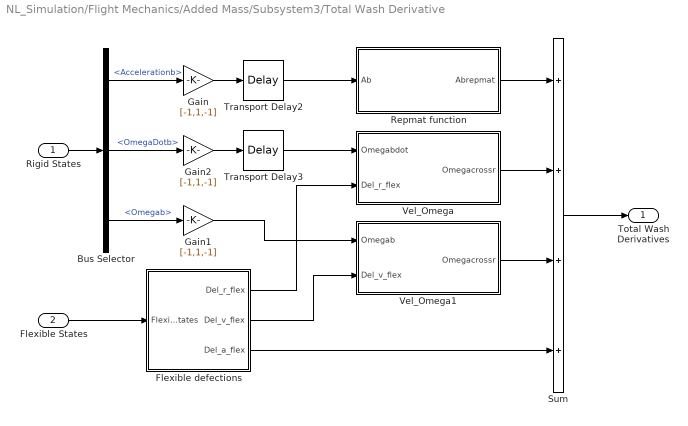
== system NL_Simulation/Flight Mechanics/Added Mass/Subsystem3/Total Wash Derivative ==
  Rigid States : Inport
  Flexible States : Inport  Port=2
  Bus Selector : BusSelector  OutputSignals=Accelerationb,OmegaDotb,Omegab
  Flexible defections : Subsystem
  Gain : Gain  Gain=[-1,1,-1]
  Gain1 : Gain  Gain=[-1,1,-1]
  Gain2 : Gain  Gain=[-1,1,-1]
  Repmat function : MATLAB Function  TreatAsAtomicUnit=on  mask{NumPanels=AC.Aero.NumPanels}
      mask prompts: NumPanels "Number of Panels"
      mask init:
      | % NumPanels = 888;
  Sum : Sum  Inputs=++++
  Transport Delay2 : TransportDelay  DelayTime=0.001  PadeOrder=2
  Transport Delay3 : TransportDelay  DelayTime=0.001  PadeOrder=2
  Vel_Omega : Subsystem
  Vel_Omega1 : Subsystem
  Total Wash Derivatives : Outport
  wires:
  Rigid States/1 -> Bus Selector/1
  Bus Selector/1 -> Gain/1  "<Accelerationb>"
  Vel_Omega/1(Omegacrossr) -> Sum/2
  Gain2/1 -> Transport Delay3/1
  Flexible States/1 -> Flexible defections/1(Flexible States)
  Sum/1 -> Total Wash Derivatives/1
  Repmat function/1(Abrepmat) -> Sum/1
  Bus Selector/2 -> Gain2/1  "<OmegaDotb>"
  Flexible defections/2(Del_v_flex) -> Vel_Omega1/2(Del_v_flex)
  Vel_Omega1/1(Omegacrossr) -> Sum/3
  Flexible defections/1(Del_r_flex) -> Vel_Omega/2(Del_r_flex)
  Gain/1 -> Transport Delay2/1
  Flexible defections/3(Del_a_flex) -> Sum/4
  Bus Selector/3 -> Gain1/1  "<Omegab>"
  Gain1/1 -> Vel_Omega1/1(Omegab)
  Transport Delay2/1 -> Repmat function/1(Ab)
  Transport Delay3/1 -> Vel_Omega/1(Omegabdot)

== system NL_Simulation/Force and Moment /Aerodynamic Model/Steady Aerodynamics/N_hat ==
  note: The effect of flexible deflections on normal vectors are calculated. The resulting normal vectors are then rotated by control surface deflection angles
  CS : Inport
  Flexible States : Inport  Port=2
  Bus Selector : BusSelector  OutputSignals=EtaFlex
  Bus Selector1 : BusSelector  OutputSignals=CS Pos
  CS effects on normal vectors : Subsystem
  Mux : Mux  Inputs=2
  Nhat_eta_all : Constant  Value=AC.Aero.Nhat_eta_all
  Normalization : dspmathops/Normalization  NormType=2-norm  Bias=1e-10  NormOver=Each column  Dimension=1  roundingMode=Floor  overflowMode=off  accumDataTypeStr=Inherit: Same as product output  accumLastDataTypeStr=Inherit: Same as product output  outputDataTypeStr=Inherit: Same as product output  outputMin=[]  outputMax=[]  outputLastDataTypeStr=Inherit: Same as product output
      settings: SourceProductName=DSP System Toolbox
  Product : Product  Multiplication=Matrix(*)
  Reshape : Reshape  OutputDimensionality=Customize  OutputDimensions=[3,AC.Aero.NumPanels]
  Reshape1 : Reshape  OutputDimensionality=Column vector (2-D)
  one : Constant
  Nhat : Outport
  wires:
  Flexible States/1 -> Bus Selector/1
  Product/1 -> Reshape/1
  Nhat_eta_all/1 -> Product/1
  CS/1 -> Bus Selector1/1
  Bus Selector1/1 -> CS effects on normal vectors/1(CS Pos)  "<CS Pos>"
  CS effects on normal vectors/1(Nhat) -> Nhat/1
  Reshape/1 -> Normalization/1
  Normalization/1 -> CS effects on normal vectors/2(Nhat_Flex)
  Bus Selector/1 -> Mux/2  "<EtaFlex>"
  one/1 -> Mux/1
  Mux/1 -> Reshape1/1
  Reshape1/1 -> Product/2

== system NL_Simulation/Force and Moment /Aerodynamic Model/Steady Aerodynamics/Normal Wash ==
  note: Take the dot product of the Total Wash to obtain the required Normal Wash. This results in the internal normal wash produced by the vortices
  Nhat : Inport
  Total Wash : Inport  Port=2
  Product : Product
  Sum : Sum  Inputs=+  CollapseMode=Specified dimension
  Transpose : Math  Operator=transpose  SaturateOnIntegerOverflow=on
  Normal Wash : Outport
  wires:
  Nhat/1 -> Product/1
  Total Wash/1 -> Product/2
  Product/1 -> Sum/1
  Sum/1 -> Transpose/1
  Transpose/1 -> Normal Wash/1
